simulink model "Controllers"  (R2023a)
settings: Solver=ode1  StartTime=0.0  StopTime=2  FixedStep=0.002  RelTol=1e-3  EnableMultiTasking=on
PostLoadFcn:
  | qc_set_target_type(getConfigSet(bdroot, 'QUARC Default Target Configuration'));
values from neighbouring files (symbols this model uses):
  A = [1 0 0 0 0.0147199567439 0.494235215112 0.00522092157741 0.491281537416 0.0846349923033 7.9640363337 0.847837602356 -15.2382982691 ... (16 elements, 4x4)]    [sysest09c_trick_fake.mat]
  Aeq = Gamma_z(end-nz+1:end,:)-Gamma_z(end-2*nz+1:end-nz,:)    [main.m]    (also in sysest09c_trick_fake.mat = [2.33147876005e-12 3.05027002175e-11 -1.39065442029e-12 -1.0)
  Azbar = zeros((N+1)*nqz,(N+1)*nz)    [main.m]    (also in sysest09c_trick_fake.mat = [])
  B = [0.00785227289808 0.752153518559 -0.00776434946027 -0.730614601908]    [sysest09c_trick_fake.mat]
  bubar = zeros(N*nqu,1)    [main.m]    (also in sysest09c_trick_fake.mat = [5 5 5 5 5 5 5 5 5 5 5 5 ... (300 elements, 300x1)])
  bzbar = zeros((N+1)*nqz,1)    [main.m]    (also in sysest09c_trick_fake.mat = [])
  C = [1  0  0  0; 0  0  1  0]    [sysest09c_trick_fake.mat]
  Gamma_y = [0 0 0.00785227289808 -0.00776434946027 0.0178205046293 -0.0164835775748 0.0198812620775 -0.0149072785302 0.0184337517661 -0.0075847210105 0.0165272112015 0.00137739075354 ... (45300 elements, 302x150)]    [sysest09c_trick_fake.mat]
  H = 0.5*(H+H')    [main.m]    (also in sysest09c_trick_fake.mat = [1394.41630764 1288.94729997 1281.54056458 1272.6112048 1262)
  Lambda_y = [1 0 1 0 1 0 1 0 1 0 1 0 ... (1208 elements, 302x4)]    [sysest09c_trick_fake.mat]
  Lambda_z = [1 0 0 0 1 0 0 0 1 0 0 0 ... (2416 elements, 604x4)]    [sysest09c_trick_fake.mat]
  N = 7    [main.m]    (also in sysest09c_trick_fake.mat = 150)
  nu = size(B,2)    [main.m]    (also in sysest09c_trick_fake.mat = 1)
  nz = size(A,1)    [main.m]    (also in sysest09c_trick_fake.mat = 4)
  Qbar = zeros((N+1)*ny)    [main.m]    (also in sysest09c_trick_fake.mat = [10000 10000 0 0 0 0 0 0 0 0 0 0 ... (91204 elements, 302x30)
  sysest_ct = d2c(sysest)    [main.m]
  v_a_max = Vbar    (= 5)    [main.m]    (also in sysest09c_trick_fake.mat)
  Yref = zeros((N+1)*ny,1)    [main.m]    (also in sysest09c_trick_fake.mat = [0.523598775598 0 0.523598775598 0 0.523598775598 0 0.523598)
undefined symbols (not defined in the file or in its folder): HIL, Kp, qc_get_step_size, sigbuilder_block, Ti
libraries: simulink_extras x7, quarc_library x4, cstblocks x1
settings Model: SimulationMode=external  ExtModeTrigDuration=5000  Creator=CFulford  LastModifiedBy=alpre
settings SolverCC: AlgebraicLoopSolver=TrustRegion  PositivePriorityOrder=on
settings DataIOCC: LimitDataPoints=on  SaveFormat=Array  SignalLoggingSaveFormat=ModelDataLogs  ReturnWorkspaceOutputs=off
settings OptimizationCC: ReuseModelBlockBuffer=off  ExpressionDepthLimit=2147483647  InitFltsAndDblsToZero=on  LifeSpan=inf
settings DebuggingCC: SaveWithParameterizedLinksMsg=none  UnderspecifiedInitializationDetection=Classic  MergeDetectMultiDrivingBlocksExec=none  SolverPrmCheckMsg=warning  MultiTaskDSMMsg=warning  MultiTaskCondExecSysMsg=none  FcnCallInpInsideContextMsg=warning  UnconnectedInputMsg=warning  UnconnectedOutputMsg=warning  UnconnectedLineMsg=warning  StateNameClashWarn=warning  SFUnexpectedBacktrackingDiag=warning  SFNoUnconditionalDefaultTransitionDiag=warning  SFExecutionAtInitializationDiag=none  ArithmeticOperatorsInVariantConditions=warning
settings HardwareCC: ProdBitPerPointer=32  ProdBitPerSizeT=32  ProdBitPerPtrDiffT=32  ProdLargestAtomicFloat=None  ProdIntDivRoundTo=Undefined  ProdEndianess=Unspecified  ProdWordSize=32  ProdHWDeviceType=32-bit Generic
settings ModelReferenceCC: EnableRefExpFcnMdlSchedulingChecks=on  PropagateSignalLabelsOutOfModel=off
settings SFSimCC: SimUseLocalCustomCode=off  CustomCodeUndefinedFunction=UseInterfaceOnly
settings RTWCC: Description=QUARC Win64 Target  SystemTargetFile=quarc_win64.tlc  TemplateMakefile=quarc_default_tmf  RTWUseLocalCustomCode=off  DLArmComputeVersion=19.05
settings CodeAppCC: StateflowObjectComments=on
settings STFCustomTargetCC: TargetPreCompLibLocation=C:\PROGRA~3\QUARC\lib\2019b\win64\release  TargetLangStandard=C89/C90 (ANSI)  CombineOutputUpdateFcns=on  CPPClassGenCompliant=on  GRTInterface=off  UseToolchainInfoCompliant=off  SystemTargetFile=quarc_win64.tlc
settings GRTTargetCC: TargetPreCompLibLocation=C:\PROGRA~3\QUARC\lib\2019b\win64\release  TargetLangStandard=C89/C90 (ANSI)  ParMdlRefBuildCompliant=off  CompOptLevelCompliant=off  MatFileLogging=off  UseToolchainInfoCompliant=off  ExtMode=on  ExtModeMexFile=quarc_comm
settings ConfigComp: CovMetricSettings=dw  CovSaveCumulativeToWorkspaceVar=on  CovSaveSingleToWorkspaceVar=on  CovExternalEMLEnable=off  CovSFcnEnable=off

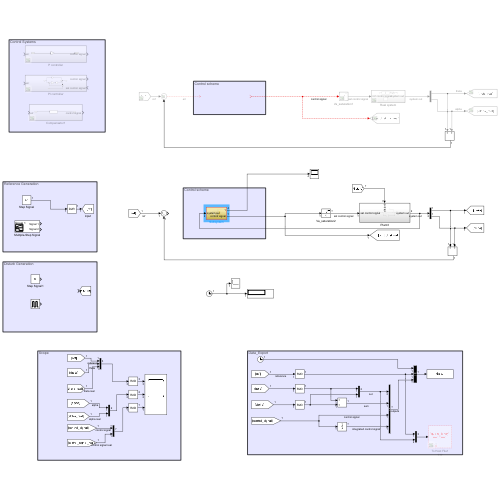
[thumbnail: Simulink's stored preview of the top-level diagram]
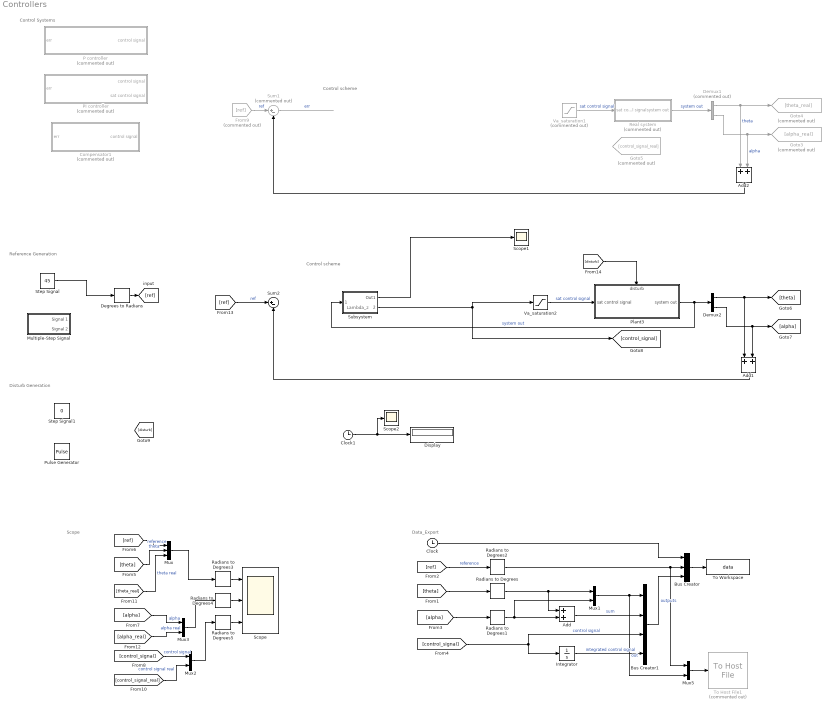
== system Controllers ==
  note: Lambda_z
  note: Reference Generation
  note: Disturb Generation
  note: Data_Export
  note: Scope
  note: Control scheme
  note: Control Systems
  note: Control scheme
  Add : Sum
  Add1 : Sum
  Add2 : Sum
  Bus Creator : BusCreator  Inputs=3
  Bus Creator1 : BusCreator  Inputs=4
  Clock : Clock
  Clock1 : Clock
  Compensator1 : Subsystem  Commented=on
  Degrees to Radians : simulink_extras/Transformations/Degrees to Radians
  Demux1 : Demux  Commented=on  Outputs=2
  Demux2 : Demux  Outputs=2
  Display : Display
  From9 : From  Commented=on  GotoTag=ref
  Goto3 : Goto  Commented=on  GotoTag=alpha_real
  Goto4 : Goto  Commented=on  GotoTag=theta_real
  Goto5 : Goto  Commented=on  GotoTag=control_signal_real
  Integrator : Integrator
  Multiple-Step Signal : Subsystem  Tag=STV Subsys  LoadFcn=sigbuilder_block('load');  StartFcn=sigbuilder_block('start');  StopFcn=sigbuilder_block('stop');  ClipboardFcn=sigbuilder_block('clipboard');  mask(Sigbuilder block){tuvar=[0:10]}
      mask help: Simulink:masks:SigbuilderBlock_MD
      mask init:
      | if ~strcmp(get_param(bdroot(gcbh),'SimulationStatus'),'stopped') tuvar = sigbuilder_block('maskInit'); end
      settings: CopyFcn=sigbuilder_block('copy');  DeleteFcn=sigbuilder_block('delete');  ModelCloseFcn=sigbuilder_block('modelClose');  PreSaveFcn=sigbuilder_block('preSave');  PauseFcn=sigbuilder_block('pause');  ContinueFcn=sigbuilder_block('continue');  NameChangeFcn=sigbuilder_block('namechange');  OpenFcn=sigbuilder_block('open',[6 30 1428 681.75 ]);  CloseFcn=sigbuilder_block('close');
      mask Display: plot(0, 0, 100, 100,[2, 2, 32, 32, 2], [68, 8, 8, 68, 68],[32, 2], [38, 38], [32, 19, 2],[53, 60, 44], [32, 17, 17, 2],[16, 16, 31, 31]);txt = getActiveGroup(gcbh);text(2, 100, txt,'verticalAlignment', 'top');
  Mux : Mux  Inputs=3
  Mux{1..3,5} (4 alike) : Mux  Inputs=2
  P controller : Subsystem  Commented=on
  PI controller : Subsystem  Commented=on
      settings: PortSchema="{\"entries\":[{\"content\":{\"sides\":[{\"content\":{\"connectorIds\":[\"In1\"]},\"type\":\"ConnectorPlacement.EquallySpacedRectSide\",\"uuid\":\"7217c107-8941-41d6-876d-785730e7c545\"},{\"content\":{\"connectorIds\":[\"Out1\",\"In2\"],\"side\":\"RIGHT\"},\"type\":\"ConnectorPlacement.EquallySpacedRectSide\",\"uuid\":\"8f4f3268-96a8-4465-82c6-7649ba2b4d82\"},{\"content\":{\"connectorIds\":[],\"side\":\"TOP\"},\"type\":\"ConnectorPlacement.EquallySpacedRectSide\",\"uuid\":\"2867d623-f00e-4653-a247-c097ef3a497d\"}]},\"type\":\"ConnectorPlacement.EquallySpacedConnector\",\"uuid\":\"1846d293-9aed-4872-b7e0-e51cb20c3863\"}],\"packageUris\":[\"http://schema.mathworks.com/mf0/Connector/R2020b\"],\"version\":\"1.0\"}"
  Plant3 : Subsystem
      settings: PortSchema="{\"entries\":[{\"content\":{\"sides\":[{\"content\":{\"connectorIds\":[\"In1\"]},\"type\":\"ConnectorPlacement.EquallySpacedRectSide\",\"uuid\":\"cdc36ef1-b9aa-4793-8815-08646de90a91\"},{\"content\":{\"connectorIds\":[\"Out1\"],\"side\":\"RIGHT\"},\"type\":\"ConnectorPlacement.EquallySpacedRectSide\",\"uuid\":\"c826576a-106c-43df-aaf0-aa674a969d04\"},{\"content\":{\"connectorIds\":[\"In2\"],\"side\":\"TOP\"},\"type\":\"ConnectorPlacement.EquallySpacedRectSide\",\"uuid\":\"d2200aa9-f6c9-47e5-a9d0-498ec6850ca3\"}]},\"type\":\"ConnectorPlacement.EquallySpacedConnector\",\"uuid\":\"4474187f-41f3-4590-923f-8ea1970bc9fc\"}],\"packageUris\":[\"http://schema.mathworks.com/mf0/Connector/R2020b\"],\"version\":\"1.0\"}"
  Pulse Generator : DiscretePulseGenerator  PulseType=Time based  Period=10  PulseWidth=5
  Radians to Degrees{,1..5} (6 alike) : simulink_extras/Transformations/Radians to Degrees
  Real system : Subsystem  Commented=on
  Scope : Scope  NumInputPorts=3
  Scope1 : Scope
  Scope2 : Scope
  Step Signal : Constant  Value=45
  Step Signal1 : Constant  Value=0
  Subsystem : Subsystem
  Sum1 : Sum  Commented=on  Inputs=|+-
  Sum2 : Sum  Inputs=|+-
  To Host File1 : quarc_library/Sinks/To Host/To Host File  Commented=on  file_name=Sine tests\Sine_24_in_theta_alpha.mat  variable_name=data  decimation=1  sample_time=-1  file_format=MAT-file v.4  options=No header or footer  append=off  final_file_name=Sine tests\Sine_24_in_theta_alpha.mat  bitrate=2000000
  To Workspace : ToWorkspace  VariableName=data  SampleTime=-1
  Va_saturation1 : Saturate  Commented=on  UpperLimit=v_a_max  LowerLimit=-v_a_max
  Va_saturation2 : Saturate  UpperLimit=v_a_max  LowerLimit=-v_a_max
  wires:
  Radians to Degrees3/1 -> Scope/1
  Radians to Degrees4/1 -> Scope/2
  Sum1/1 -> ?  "err"
  Mux3/1 -> Radians to Degrees4/1
  ? -> Va_saturation1/1, Goto5/1  "control signal"
  Radians to Degrees2/1 -> Mux5/1, Bus Creator/2
  [control_signal] -> Integrator/1, Bus Creator1/3  "control signal"
  [alpha] -> Radians to Degrees1/1
  Bus Creator1/1 -> Bus Creator/3  "outputs"
  Clock/1 -> Bus Creator/1
  [disturb] -> Plant3/2(disturb)
  Demux2/1 -> Add1/1, [theta]
  Mux/1 -> Radians to Degrees3/1
  [ref] -> Sum2/1  "ref"
  Radians to Degrees/1 -> Add/1, Mux1/1
  [control_signal_real] -> Mux2/2  "control signal real"
  Add/1 -> Bus Creator1/2  "sum"
  [theta] -> Radians to Degrees/1
  [ref] -> Radians to Degrees2/1  "reference"
  Integrator/1 -> Bus Creator1/4  "integrated control signal"
  Bus Creator/1 -> To Workspace/1
  [alpha_real] -> Mux3/2  "alpha real"
  Mux5/1 -> To Host File1/1
  Demux1/1 -> Add2/1, Goto4/1  "theta"
  Real system/1(system out) -> Demux1/1  "system out"
  [theta_real] -> Mux/3  "theta real"
  Va_saturation2/1 -> Plant3/1(sat control signal)  "sat control signal"
  From9/1 -> Sum1/1  "ref"
  Radians to Degrees1/1 -> Add/2, Mux1/2
  Demux1/2 -> Goto3/1, Add2/2  "alpha"
  Plant3/1(system out) -> Subsystem/1(system out), Demux2/1  "system out"
  [control_signal] -> Mux2/1  "control signal"
  Degrees to Radians/1 -> [ref]
  Radians to Degrees5/1 -> Scope/3
  [ref] -> Mux/1  "reference"
  Mux2/1 -> Radians to Degrees5/1
  Va_saturation1/1 -> Real system/1(sat control signal)  "sat control signal"
  [alpha] -> Mux3/1  "alpha"
  Mux1/1 -> Mux5/2, Bus Creator1/1  "out"
  [theta] -> Mux/2  "theta"
  Demux2/2 -> Add1/2, [alpha]
  Step Signal/1 -> Degrees to Radians/1
  Add1/1 -> Sum2/2
  Add2/1 -> Sum1/2
  Subsystem/2(control signal) -> [control_signal], Va_saturation2/1
  Subsystem/1(Out1) -> Scope1/1
  Clock1/1 -> Scope2/1, Display/1

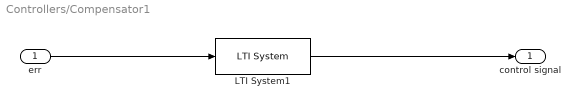
== system Controllers/Compensator1 ==
  err : Inport
  LTI System1 : cstblocks/LTI System  sys=controller  IC=[]
  control signal : Outport
  wires:
  LTI System1/1 -> control signal/1
  err/1 -> LTI System1/1

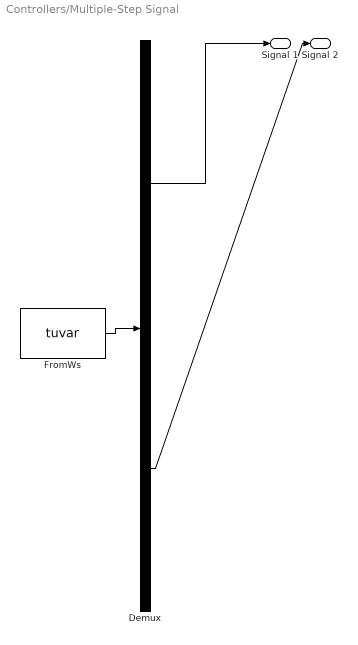
== system Controllers/Multiple-Step Signal ==
  Demux : Demux  Tag=STV Demux  Outputs=2
      settings: DisplayOption=none
  FromWs : FromWorkspace  Tag=STV FromWs  VariableName=tuvar
      SigBuilderData=|
      | common.afterFinalStr = 'Extrapolate'
      | common.sampleTime = 0
      | dataSet.timeRange = [0 10]
      | dataSet.name = 'Group 1'
      | sbobj.Groups.Name = 'Group 1'
      | sbobj.Groups.Signals(1).Name = 'Signal 1'
      | sbobj.Groups.Signals(1).XData = [0 1 1 3 3 7 7 8.5 8.5 10]
      | sbobj.Groups.Signals(1).YData = [0.005 0.005 40 40 -30 -30 0 0 23 23]
      | sbobj.Groups.Signals(2).Name = 'Signal 2'
      | sbobj.Groups.Signals(2).XData = [0 1 1 1.52 10]
      | sbobj.Groups.Signals(2).YData = [0 0 -40 -40 -40]
  Signal 1 : Outport  Tag=STV Outport
  Signal 2 : Outport  Tag=STV Outport  Port=2
  wires:
  Demux/1 -> Signal 1/1
  FromWs/1 -> Demux/1
  Demux/2 -> Signal 2/1

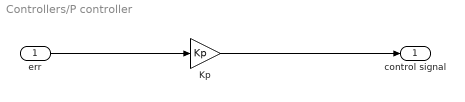
== system Controllers/P controller ==
  err : Inport
  Kp : Gain  Gain=Kp
  control signal : Outport
  wires:
  err/1 -> Kp/1
  Kp/1 -> control signal/1

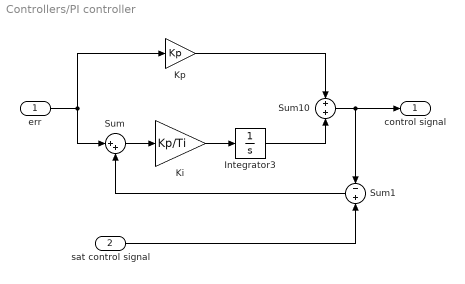
== system Controllers/PI controller ==
  err : Inport
  sat control signal : Inport  Port=2
  Integrator3 : Integrator
  Ki : Gain  Gain=Kp/Ti
  Kp : Gain  Gain=Kp
  Sum : Sum  Inputs=|++
  Sum1 : Sum  Inputs=-+
  Sum10 : Sum
  control signal : Outport
  wires:
  err/1 -> Sum/1, Kp/1
  Ki/1 -> Integrator3/1
  Sum10/1 -> control signal/1, Sum1/1
  Integrator3/1 -> Sum10/2
  Kp/1 -> Sum10/1
  Sum/1 -> Ki/1
  sat control signal/1 -> Sum1/2
  Sum1/1 -> Sum/2

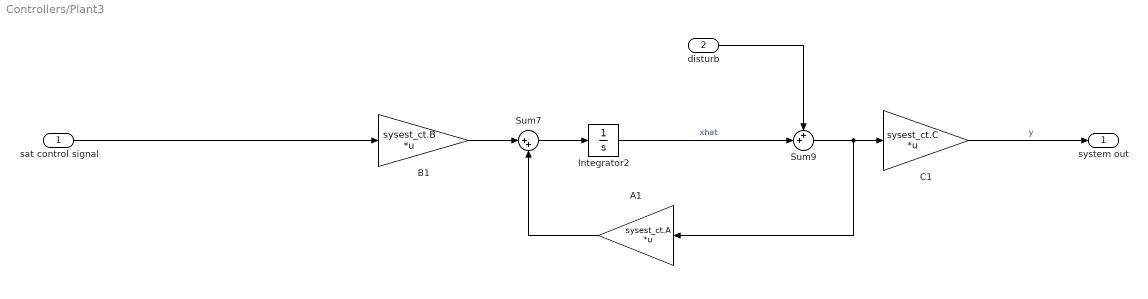
== system Controllers/Plant3 ==
  sat control signal : Inport
  disturb : Inport  Port=2
  A1 : Gain  Gain=sysest_ct.A  Multiplication=Matrix(K*u)
  B1 : Gain  Gain=sysest_ct.B  Multiplication=Matrix(K*u)
  C1 : Gain  Gain=sysest_ct.C  Multiplication=Matrix(K*u)
  Integrator2 : Integrator
  Sum7 : Sum  Inputs=|++
  Sum9 : Sum  Inputs=++|
  system out : Outport
  wires:
  Sum7/1 -> Integrator2/1
  disturb/1 -> Sum9/1
  B1/1 -> Sum7/1
  Integrator2/1 -> Sum9/2  "xhat"
  C1/1 -> system out/1  "y"
  A1/1 -> Sum7/2
  Sum9/1 -> A1/1, C1/1
  sat control signal/1 -> B1/1

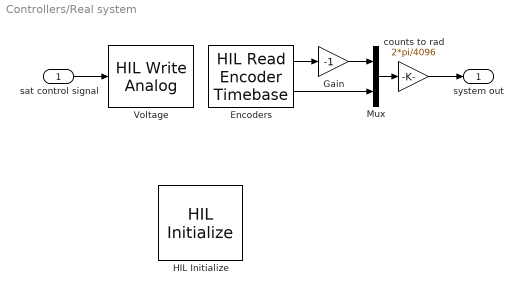
== system Controllers/Real system ==
  sat control signal : Inport
  Encoders : quarc_library/Data Acquisition/Generic/Timebases/HIL Read Encoder Timebase  object_name=HIL-1  clock=0  channels=[0:1]  samples_in_buffer=max(ceil(1/qc_get_step_size), 1)  active=on  vector_output=off  data_type_mode=Inherit via back propagation  data_type=double
  Gain : Gain  Gain=-1
  HIL Initialize : quarc_library/Data Acquisition/Generic/Configuration/HIL Initialize  Priority=-99  object_name=HIL-1  board_type=q2_usb  board_number=0  board_options=d0=digital;d1=digital;led=auto;update_rate=normal;decimation=1  exclusive=off  active=off  hardware_clocks=[0]  clock_modes=[]  initial_clock_frequencies=[]  set_clock_params_at_start=off  set_clock_params_at_switch_in=off  set_clock_frequencies_at_start=off  set_clock_frequencies_at_switch_in=off  analog_input_channels=[0:1]  analog_input_configurations=[]  analog_input_maximums=10  analog_input_minimums=-10  set_analog_input_params_at_start=on  set_analog_input_params_at_switch_in=off  analog_output_channels=[0:1]  analog_output_maximums=10  analog_output_minimums=-10  initial_analog_outputs=[0]  final_analog_outputs=[0]  watchdog_analog_outputs=0  set_analog_output_params_at_start=on  set_analog_output_params_at_switch_in=off  set_analog_outputs_at_start=on  set_analog_outputs_at_switch_in=off  set_analog_outputs_at_terminate=on  set_analog_outputs_at_switch_out=off  set_analog_outputs_on_watchdog=off  digital_input_channels=[]  digital_output_channels=[]  digital_output_configuration=[]  initial_digital_outputs=[1]  final_digital_outputs=[1]  watchdog_digital_outputs=[1]  set_digital_output_params_at_start=off  set_digital_output_params_at_switch_in=off  set_digital_outputs_at_start=on  set_digital_outputs_at_switch_in=off  set_digital_outputs_at_terminate=on  set_digital_outputs_at_switch_out=off  set_digital_outputs_on_watchdog=off  encoder_channels=[0:1]  quadrature=[4]  encoder_filter_frequency=[]  initial_encoder_counts=[0]  set_encoder_params_at_start=on  set_encoder_params_at_switch_in=off  set_encoder_counts_at_start=on  set_encoder_counts_at_switch_in=off  pwm_channels=[]  pwm_modes=[0]  pwm_frequency=1/0.020  pwm_configuration=[]  pwm_alignment=[]  pwm_polarity=[]  pwm_leading_deadband=[]  pwm_trailing_deadband=[]  initial_pwm_outputs=[0]  final_pwm_outputs=[0]  watchdog_pwm_outputs=[0]  set_pwm_params_at_start=on  set_pwm_params_at_switch_in=off  set_pwm_outputs_at_start=on  set_pwm_outputs_at_switch_in=off  set_pwm_outputs_at_terminate=on  set_pwm_outputs_at_switch_out=off  set_pwm_outputs_on_watchdog=off  other_output_channels=[]  initial_other_outputs=[]  final_other_outputs=[]  watchdog_other_outputs=[]  set_other_outputs_at_start=off  set_other_outputs_at_switch_in=off  set_other_outputs_at_terminate=off  set_other_outputs_at_switch_out=off  set_other_outputs_on_watchdog=off
  Mux : Mux  Inputs=2
  Voltage : quarc_library/Data Acquisition/Generic/Immediate I//O/HIL Write Analog  object_name=HIL-1  channels=0  sample_time=-1  active=off  vector_input=off
  counts to rad : Gain  Gain=2*pi/4096
  system out : Outport
  wires:
  sat control signal/1 -> Voltage/1
  Encoders/1 -> Gain/1
  Encoders/2 -> Mux/2
  Mux/1 -> counts to rad/1
  Gain/1 -> Mux/1
  counts to rad/1 -> system out/1

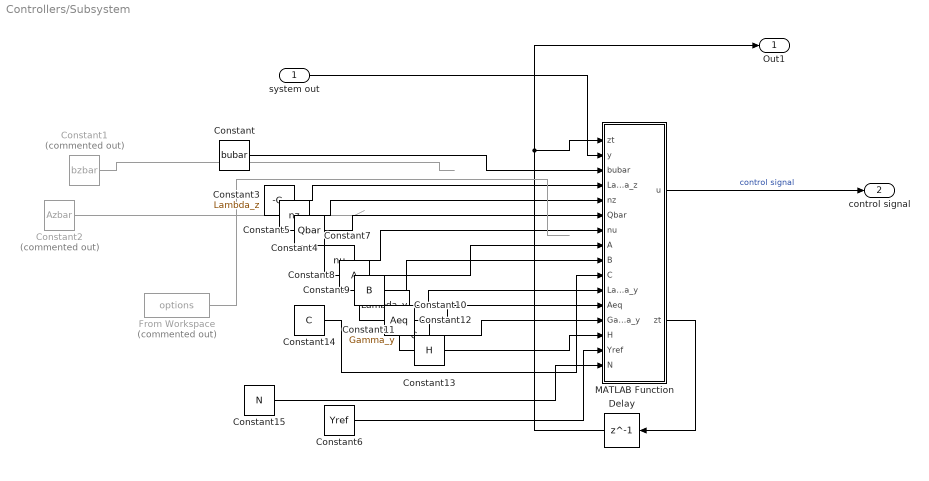
== system Controllers/Subsystem ==
  system out : Inport
  Constant : Constant  Value=bubar
  Constant1 : Constant  Commented=on  Value=bzbar
  Constant10 : Constant  Value=Lambda_y
  Constant11 : Constant  Value=Gamma_y
  Constant12 : Constant  Value=Aeq
  Constant13 : Constant  Value=H
  Constant14 : Constant  Value=C
  Constant15 : Constant  Value=N
  Constant2 : Constant  Commented=on  Value=Azbar
  Constant3 : Constant  Value=Lambda_z
  Constant4 : Constant  Value=nz
  Constant5 : Constant  Value=Qbar
  Constant6 : Constant  Value=Yref
  Constant7 : Constant  Value=nu
  Constant8 : Constant  Value=A
  Constant9 : Constant  Value=B
  Delay : Delay  DelayLength=1  InitialCondition=[0 0 0 0]'
  From Workspace : FromWorkspace  Commented=on  VariableName=options
  MATLAB Function : MATLAB Function  TreatAsAtomicUnit=on
  Out1 : Outport
  control signal : Outport  Port=2
  wires:
  Delay/1 -> Out1/1, MATLAB Function/1("zt ")
  MATLAB Function/1(u) -> control signal/1  "control signal"
  MATLAB Function/2(zt) -> Delay/1
  system out/1 -> MATLAB Function/2(y)
  Constant/1 -> MATLAB Function/3(bubar)
  Constant1/1 -> ?
  Constant2/1 -> ?
  Constant3/1 -> MATLAB Function/4(Lambda_z)
  Constant4/1 -> MATLAB Function/5(nz)
  Constant5/1 -> MATLAB Function/6(Qbar)
  Constant7/1 -> MATLAB Function/7(nu)
  Constant8/1 -> MATLAB Function/8(A)
  Constant9/1 -> MATLAB Function/9(B)
  Constant10/1 -> MATLAB Function/11(Lambda_y)
  Constant12/1 -> MATLAB Function/12(Aeq)
  Constant11/1 -> MATLAB Function/13(Gamma_y)
  Constant13/1 -> MATLAB Function/14(H)
  From Workspace/1 -> ?
  Constant6/1 -> MATLAB Function/15(Yref)
  Constant14/1 -> MATLAB Function/10(C)
  Constant15/1 -> MATLAB Function/16(N)

== matlab function Controllers/Subsystem/MATLAB Function ==
  data: zt input; u output; zt output; y input; bubar input; Lambda_z input; nz input; Qbar input; nu input; A input; B input; C input; Lambda_y input; Aeq input; Gamma_y input; H input; Yref input; N input
function [u , zt]   = fcn(zt, y, bubar, Lambda_z, nz, Qbar, nu, A, B,C, Lambda_y ,Aeq, Gamma_y , H,Yref, N )
%function [u , zt]   = fcn(zt, y, bubar, bzbar, Azbar, Lambda_z, nz, Qbar,  options, nu, A, B, Lambda_y ,Aeq, Gamma_y , H )
U = zeros(N,1);
u = 0;
zt = zeros(4,1);
zt(1) = y(1);
zt(3) = y(2);
options = optimoptions('quadprog','Algorithm','active-set');
%options = optimoptions('quadprog','Algorithm','trust-region-reflective');
[row, col] = size(H);
x0 = zeros(row, 1);

%bineq                               =   [bubar;bzbar-Azbar*Lambda_z*zt];
bineq                               =   [bubar];%;bzbar-Azbar*Lambda_z*zt];
beq                                 =   -(Lambda_z(end-nz+1:end,:)-Lambda_z(end-2*nz+1:end-nz,:))*zt;
f                                   =   zt'*Lambda_y'*Qbar*Gamma_y-Yref'*Qbar*Gamma_y;

U                                   =   quadprog(H,f,[],[],Aeq,beq,[],[],x0,options);

zt  =   A*zt+B*U(1:nu,1);
%zt                                 =   Zsim_MPC((ind-1)*nz+1:ind*nz,1);

%u = U(1:nu,1);
u = U(1,1);

end
